simulink model "testrig_susp_knc"  (R2026a)
settings: Solver=ode23t  StopTime=309  MaxStep=0.1  AbsTol=1e-3  EnableMultiTasking=on
PostLoadFcn:
  | Maneuver = MDatabase.KnC.FSAE_Achilles;
  | Visual = sm_car_param_visual('default');
values from neighbouring files (symbols this model uses):
  Vehicle = sm_car_vehcfg_setPeopleOnOff(Vehicle,[0 0 0 0 0],'SuspA1')    [testrig_susp_knc_results.m]
undefined symbols (not defined in the file or in its folder): Axle1D, AxleIn, Init, RaceFix, RaceSpin, X, Y, Z
libraries: fl_lib x12, sm_lib x8, sm_car_testrig_utilities_lib x6, nesl_utility x5, Damper_Element x2, Linkage x1
CloseFcn:
  | clear simlog_sm_car_testrig_quarter_car
  | clear logsout_sm_car_testrig_quarter_car
  | Maneuver = MDatabase.Skidpad.FSAE_Achilles;
Description:
  | Half Car Testrig, Pullrod
  | 
  | Copyright 2021-2024 The MathWorks, Inc.
settings Model: Creator=smiller  LastModifiedBy=andrei
settings SolverCC: MinimalZcImpactIntegration=on
settings DataIOCC: SignalLoggingName=logsout_sm_car_testrig_quarter_car
settings DebuggingCC: ReadBeforeWriteMsg=DisableAll  WriteAfterWriteMsg=DisableAll  WriteAfterReadMsg=DisableAll  MultiTaskDSMMsg=none
settings SFSimCC: SFSimEcho=off
settings SimscapeCC: SimscapeNominalValues="[{\"value\":\"1\",\"unit\":\"A\"},{\"value\":\"1\",\"unit\":\"bar\"},{\"value\":\"1\",\"unit\":\"cm^2\"},{\"value\":\"1\",\"unit\":\"cm^3/s\"},{\"value\":\"1\",\"unit\":\"kJ/kg\"},{\"value\":\"1\",\"unit\":\"kW\"},{\"value\":\"1\",\"unit\":\"l\"},{\"value\":\"1\",\"unit\":\"N\"},{\"value\":\"1\",\"unit\":\"N*m\"},{\"value\":\"1\",\"unit\":\"V\"}]"  SimscapeLogSimulationStatistics=on  SimscapeLogName=simlog_sm_car_testrig_quarter_car  SimscapeLogLimitData=off  SimscapeOperatingPoint=op
settings DiagnosticsConfigSet: SimMechanicsUnconnectedFramePorts=none  SimMechanicsConflictingReferenceFrames=none
settings ExplorerConfigSet: InternalSimMechanicsExplorerSettings=|
  | <ExplorerConfiguration>
  | 
  |   <canonicalview>default</canonicalview>
  | 
  |   <TilePanel>
  |     <TileInfo>
  |       <Tiles Columns="1" Count="1" Height="1112" Rows="1" Width="2985">
  |         <Row Weight="1"/>
  |         <Column Weight="1"/>
  |         <Tile Height="1" Width="1" X="0" Y="0"/>
  |       </Tiles>
  |     </TileInfo>
  |     <SceneInfo>
  |       <SceneViewer>
  |         <IsThisViewStd>
  |           <IsStandardView>off</IsStandardView>
  |           <StandardViewName>Front</StandardViewName>
  |         </IsThisViewStd>
  |         <BGColor>
  |           <R>1</R>
  |           <G>1</G>
  |           <B>1</B>
  |           <A>1</A>
  |         </BGColor>
  |         <Camera>
  |           <DoPerspective>off</DoPerspective>
  |           <Position>
  |             <X>0.57193000000000005</X>
  |             <Y>-0.57911000000000001</Y>
  |             <Z>0.83606000000000003</Z>
  |           </Position>
  |           <Center>
  |             <X>-0.0054200000000000003</X>
  |             <Y>-0.0017600000000000001</Y>
  |             <Z>0.25871</Z>
  |           </Center>
  |           <Up>
  |             <X>-0.40824829046386302</X>
  |             <Y>0.40824829046386302</Y>
  |             <Z>0.81649658092772603</Z>
  |           </Up>
  |           <XLim>0.89132328168650055</XLim>
  |           <YLim>0.71867958298145773</YLim>
  |           <ViewLimDist>0.01</ViewLimDist>
  |         </Camera>
  |       </SceneViewer>
  |     </SceneInfo>
  |   </TilePanel>
  | 
  |   <MechEditorPanel>
  |     <GfxPanelCameraMap/>
  |     <Cameras/>
  |     <VideoCreator>
  |       <IncludeTiles>All</IncludeTiles>
  |       <IncludeTime>on</IncludeTime>
  |       <IncludeWorldFrame>off</IncludeWorldFrame>
  |       <PlaybackSpeedRatio>1</PlaybackSpeedRatio>
  |       <FrameRate>30</FrameRate>
  |       <FrameSize>auto</FrameSize>
  |       <VideoFormat>MotionJPEGAVI</VideoFormat>
  |     </VideoCreator>
  |   </MechEditorPanel>
  | 
  |   <PlaybackSettings>
  |     <PlaybackSpeedFactor>16</PlaybackSpeedFactor>
  |   </PlaybackSettings>
  | 
  | </ExplorerConfiguration>

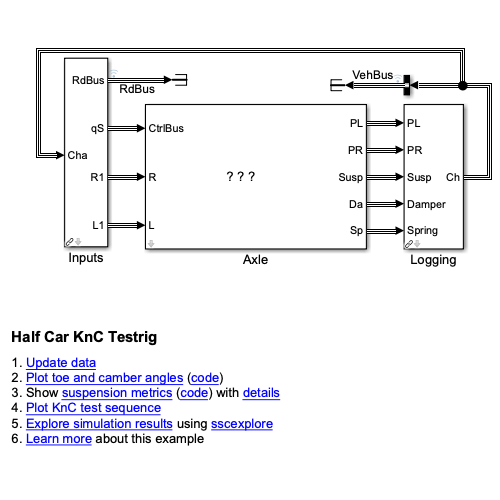
[thumbnail: Simulink's stored preview of the top-level diagram]
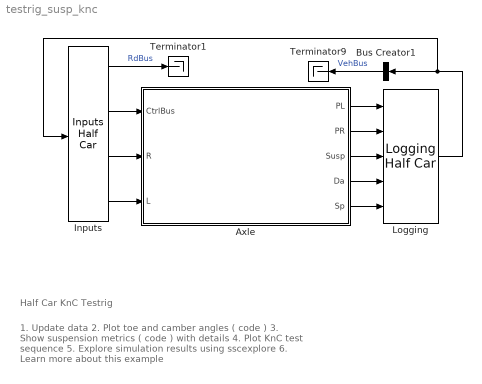
== system testrig_susp_knc ==
  note: Half Car KnC Testrig
  note: 1. Update data
      | 2. Plot toe and camber angles ( code )
      | 3. Show suspension metrics ( code ) with details
      | 4. Plot KnC test sequence
      | 5. Explore simulation results using sscexplore
      | 6. Learn more about this example
  Axle : Subsystem  mask{AxNum=Rear, Vehicle=Vehicle}
      mask prompts: AxNum "Axle"; Vehicle "Vehicle (structure)"
      mask init:
      | curblk = gcb;
      | 
      | AxNumSelection = get_param(curblk,'AxNum');
      | 
      | sWctrSet = sm_car_get_sWheelCentre(Vehicle);
      | 
      | tire_radius = sm_car_vehcfg_getTireRadius(Vehicle);
      | 
      | if strcmp(AxNumSelection,'Front')
      |     axleField = 'Axle1';
      |     suspField = 'SuspA1';
      |     tireField = 'TireA1';
      |     set_param([bdroot '/Inputs'], 'popup_steering_input', 'On');
      |     sWCtr     = sWctrSet(1,:);
      | 
      | else
      |     axleField = 'Axle2';
      |     suspField = 'SuspA2';
      |     tireField = 'TireA2';
      |     set_param([bdroot '/Inputs'], 'popup_steering_input', 'Off');
      |     sWCtr     = sWctrSet(2,:);
      | 
      | end
      | if(strcmp(Vehicle.Chassis.(suspField).class.Value,'Decoupled'))
      |     springLparam = Vehicle.Chassis.Spring.(axleField).Heave;
      |     springLclass = Vehicle.Chassis.Spring.(axleField).Heave.class.Value;
      |     springRparam = Vehicle.Chassis.Spring.(axleField).Roll;
      |     springRclass = Vehicle.Chassis.Spring.(axleField).Roll.class.Value;
      |     damperLparam = Vehicle.Chassis.Damper.(axleField).Heave;
      |     damperLclass = Vehicle.Chassis.Damper.(axleField).Heave.class.Value;
      |     damperRparam = Vehicle.Chassis.Damper.(axleField).Roll;
      |     damperRclass = Vehicle.Chassis.Damper.(axleField).Roll.class.Value;
      | else
      |     springLparam = Vehicle.Chassis.Spring.(axleField);
      |     springLclass = Vehicle.Chassis.Spring.(axleField).class.Value;
      |     springRparam = Vehicle.Chassis.Spring.(axleField);
      |     springRclass = Vehicle.Chassis.Spring.(axleField).class.Value;
      |     damperLparam = Vehicle.Chassis.Damper.(axleField);
      |     damperLclass = Vehicle.Chassis.Damper.(axleField).class.Value;
      |     damperRparam = Vehicle.Chassis.Damper.(axleField);
      |     damperRclass = Vehicle.Chassis.Damper.(axleField).class.Value;
      | end
      mask TypeOptions AxNum: Front | Rear
      mask Display:
      | curblk = gcb;
      | activeVar  = get_param([curblk '/Suspension'],'activevariant');
      | varChoices = get_param([curblk '/Suspension'],'VariantChoices');
      | 
      | varInd = find(strcmp(activeVar,{varChoices(:).Name}));
      | 
      | ActiveVarCmd = get_param(varChoices(varInd).BlockName,'MaskDisplay');
      | eval(ActiveVarCmd);
  Bus Creator1 : BusCreator  Inputs=1
  Inputs : sm_car_testrig_utilities_lib/Inputs Half Car  popup_steering_input=Off
  Logging : sm_car_testrig_utilities_lib/Logging Half Car
  Terminator1 : Terminator
  Terminator9 : Terminator
  wires:
  Bus Creator1/1 -> Terminator9/1  "VehBus"
  Logging/1 -> Inputs/1, Bus Creator1/1
  Inputs/1 -> Terminator1/1  "RdBus"
  Inputs/3 -> Axle/2(R)
  Inputs/4 -> Axle/3(L)
  Inputs/2 -> Axle/1("CtrlBus ")
  Axle/1(PL) -> Logging/1
  Axle/2(PR) -> Logging/2
  Axle/3(Susp) -> Logging/3
  Axle/4(" Da") -> Logging/4
  Axle/5(" Sp") -> Logging/5

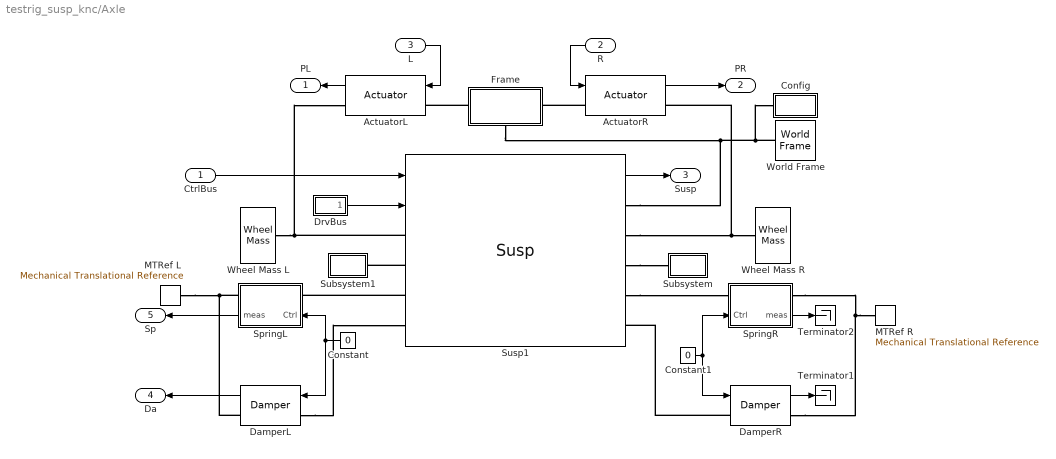
== system testrig_susp_knc/Axle ==
  "CtrlBus " : Inport
  R : Inport  Port=2
  L : Inport  Port=3
  ActuatorL : sm_car_testrig_utilities_lib/Actuator  tire_rad=tire_radius  xCPOffset=Maneuver.xCPOffset
  ActuatorR : sm_car_testrig_utilities_lib/Actuator  tire_rad=tire_radius  xCPOffset=Maneuver.xCPOffset
  Config : Subsystem
  Constant : Constant  Value=0
  Constant1 : Constant  Value=0
  DamperL : Damper_Element/Damper  VariantControl=Variant1  LabelModeActiveChoice=Nonlinear  Damper=damperLparam  VariantLabel=damperLclass
      settings: AttributesFormatString=%<ActiveVariant>
  DamperR : Damper_Element/Damper  VariantControl=Variant1  LabelModeActiveChoice=Nonlinear  Damper=damperRparam  VariantLabel=damperRclass
      settings: AttributesFormatString=%<ActiveVariant>
  DrvBus : Subsystem
  Frame : Subsystem  mask{sWctr=sWCtr}
      mask prompts: sWctr "HP Wheel Center [x y z] (m)"
      settings: PortSchema="{\"entries\":[{\"content\":{\"sides\":[{\"content\":{\"connectorIds\":[\"LConn1\"]},\"type\":\"ConnectorPlacement.EquallySpacedRectSide\",\"uuid\":\"6bafd3c1-bcc7-4e93-aea7-1b45691869cb\"},{\"content\":{\"connectorIds\":[\"RConn1\"],\"side\":\"RIGHT\"},\"type\":\"ConnectorPlacement.EquallySpacedRectSide\",\"uuid\":\"8302b8de-ad89-4cb7-8500-2e46ba409587\"},{\"content\":{\"connectorIds\":[],\"side\":\"TOP\"},\"type\":\"ConnectorPlacement.EquallySpacedRectSide\",\"uuid\":\"64bfca4e-c32f-4ac3-9207-4b63dfa53628\"},{\"content\":{\"connectorIds\":[\"RConn2\"],\"side\":\"BOTTOM\"},\"type\":\"ConnectorPlacement.EquallySpacedRectSide\",\"uuid\":\"4259e7bb-430d-411d-8823-9d547be42692\"}]},\"type\":\"ConnectorPlacement.EquallySpacedConnector\",\"uuid\":\"5df32ab5-9c2e-4acb-a8ad-c01b5f56a7cb\"}],\"packageUris\":[\"http://schema.mathworks.com/mf0/Connector/R2020b\"],\"version\":\"1.0\"}"
  MTRef L : fl_lib/Mechanical/Translational Elements/Mechanical Translational Reference
  MTRef R : fl_lib/Mechanical/Translational Elements/Mechanical Translational Reference
  SpringL : Subsystem  Variant=on  VariantControlMode=label  VariantControl=Variant1  LabelModeActiveChoice=Linear  mask(Variants for Spring){Spring=springLparam, VariantLabel=springLclass}
      mask prompts: Spring "Spring Parameters"; VariantLabel "Variant Label"
      mask help: Select option and provide parameters for spring. Option is chosen by string provided in Variant Label. The parameters for the selected option is contained in Spring data structure.
      mask init:
      | curblk = gcb;
      | 
      | % Set variant for this block 
      | set_param(curblk,'LabelModeActiveChoice',VariantLabel);
      settings: AttributesFormatString=%<ActiveVariant>
      mask Display: disp(' ')
  SpringR : Subsystem  Variant=on  VariantControlMode=label  VariantControl=Variant1  LabelModeActiveChoice=Linear  mask(Variants for Spring){Spring=springRparam, VariantLabel=springRclass}
      mask prompts: Spring "Spring Parameters"; VariantLabel "Variant Label"
      mask help: Select option and provide parameters for spring. Option is chosen by string provided in Variant Label. The parameters for the selected option is contained in Spring data structure.
      mask init:
      | curblk = gcb;
      | 
      | % Set variant for this block 
      | set_param(curblk,'LabelModeActiveChoice',VariantLabel);
      settings: AttributesFormatString=%<ActiveVariant>
      mask Display: disp(' ')
  Subsystem : Subsystem
  Subsystem1 : Subsystem
  Susp1 : Linkage/Susp  VariantControl=Variant1  LabelModeActiveChoice=Linkage  Susp=Vehicle.Chassis.(suspField)  Init=Init.(axleField)  VariantLabel=Vehicle.Chassis.(suspField).class.Value
      settings: AttributesFormatString=%<LabelModeActiveChoice>
  Terminator1 : Terminator
  Terminator2 : Terminator
  Wheel Mass L : sm_car_testrig_utilities_lib/Wheel Mass  tire_param=Vehicle.Chassis.Tire.tirFile.Value
  Wheel Mass R : sm_car_testrig_utilities_lib/Wheel Mass  tire_param=Vehicle.Chassis.Tire.tirFile.Value
  World Frame : sm_lib/Frames and Transforms/World Frame
  PL : Outport
  PR : Outport  Port=2
  Susp : Outport  Port=3
  " Da" : Outport  Port=4
  " Sp" : Outport  Port=5
  wires:
  DamperL/1 -> " Da"/1
  "CtrlBus "/1 -> Susp1/1
  DamperR/1 -> Terminator1/1
  SpringL/1(" meas") -> " Sp"/1
  SpringR/1(" meas") -> Terminator2/1
  ActuatorL/1 -> PL/1
  DrvBus/1(Out1) -> Susp1/2
  Susp1/1 -> Susp/1
  R/1 -> ActuatorR/1
  L/1 -> ActuatorL/1
  ActuatorR/1 -> PR/1
  Constant/1 -> DamperL/1, SpringL/1("Ctrl ")
  Constant1/1 -> DamperR/1, SpringR/1("Ctrl ")
  connections:
  Susp1/RConn3 -- Subsystem/LConn1
  DamperR/LConn1 -- Susp1/RConn5
  World Frame/RConn1 -- Susp1/RConn1 -- Frame/RConn2 -- Config/RConn1
  ActuatorR/RConn1 -- Susp1/RConn2 -- Wheel Mass R/RConn1
  Susp1/LConn3 -- SpringL/LConn1
  Susp1/RConn4 -- SpringR/LConn1
  MTRef L/LConn1 -- DamperL/RConn1 -- SpringL/RConn1
  Wheel Mass L/RConn1 -- Susp1/LConn1 -- ActuatorL/RConn1
  Frame/LConn1 -- ActuatorL/LConn1
  MTRef R/LConn1 -- DamperR/RConn1 -- SpringR/RConn1
  ActuatorR/LConn1 -- Frame/RConn1
  DamperL/LConn1 -- Susp1/LConn4
  Susp1/LConn2 -- Subsystem1/LConn1

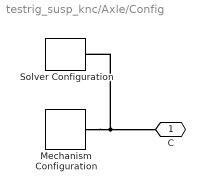
== system testrig_susp_knc/Axle/Config ==
  Mechanism Configuration : sm_lib/Utilities/Mechanism Configuration  UniformGravity=Constant  GravityVector=[0 0 -9.80665]  GravityVectorUnits=m/s^2  LinearizationDelta=0.001  JointModeTransitionNonlinearIterations=2
  Solver Configuration : nesl_utility/Solver Configuration  PhysicalDomain=network_engine_domain  SubClassName=solver  LeftPortType=input  RightPortType=generic  Tones=[]  Harmonics=[]  SimulateNoise=off  Profile=off  UseLocalSampling=off  EnableSwitchedLinearOptims=on  FrequencyDomain=off  UseCCode=off  RelTol=0.001  AbsTol=1e-06  MinStep=1e-09  ToWorkspace=off  RevertToSquareIcSolve=off  NumHomotopyIterations=100  PhasorMode=off  PhasorModeNumHarmonics=1  ConsistencySolver=NEWTON_FTOL  CanonicalOrdering=UNORDERED  OptimizeIntermediates=UNOPTIMIZED  IndexReductionMethod=DerivativeReplacement  DoDC=off  ResidualTolerance=1e-09  ConsistencyTolSource=GLOBAL  ConsistencyAbsTol=0.001  ConsistencyRelTol=0.001  ConsistencyTolFactor=0.001  UseLocalSolver=off  LocalSolverChoice=NE_BACKWARD_EULER_ADVANCER  ResolveIndetEquations=on  FunctionEvalNumThread=1  LocalSolverSampleTime=0.001  DoFixedCost=off  MaxNonlinIter=3  MaxModeIter=2  ComputeImpulses=off  ImpulseIterations=2  LinearAlgebra=Sparse  LinearAlgebraNumThread=0  EquationFormulation=NE_TIME_EF  DelaysMemoryBudget=1024  AutomaticFiltering=on  FilteringTimeConstant=0.001  PartitionStorageMethod=AS_NEEDED  PartitionMemoryBudget=1024  PartitionMethod=FAST  MultibodyUseLocalSolver=off  MultibodyLocalSolverChoice=ODE1  MultibodyLocalSolverSampleTime=0.001
  C : PMIOPort  Side=Right
  connections:
  Mechanism Configuration/RConn1 -- Solver Configuration/RConn1 -- C/RConn1

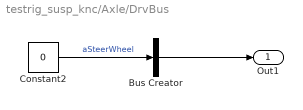
== system testrig_susp_knc/Axle/DrvBus ==
  Bus Creator : BusCreator  Inputs=1
  Constant2 : Constant  Value=0
  Out1 : Outport
  wires:
  Constant2/1 -> Bus Creator/1  "aSteerWheel"
  Bus Creator/1 -> Out1/1

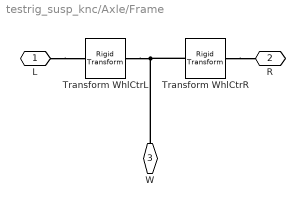
== system testrig_susp_knc/Axle/Frame ==
  Transform WhlCtrL : sm_lib/Frames and Transforms/Rigid Transform  RotationMethod=None  FollAlignAxisA=+X  BaseAlignAxisA=+Y  FollAlignAxisB=+Y  BaseAlignAxisB=+Z  RotationStandardAxis=+Z  RotationAngle=0.0  RotationAngleUnits=deg  RotationArbitraryAxis=[0 0 1]  RotationSequenceAxes=FollowerAxes  RotationSequence=XYX  RotationSequenceAngles=[0 0 0]  RotationSequenceAnglesUnits=deg  RotationMatrix=[1 0 0; 0 1 0; 0 0 1]  Quaternion=[1 0 0 0]  TranslationMethod=Cartesian  TranslationCartesianOffset=sWctr  TranslationCartesianOffsetUnits=m  TranslationStandardAxis=+Z  TranslationStandardOffset=0  TranslationStandardOffsetUnits=m  TranslationROffset=0  TranslationROffsetUnits=m  TranslationThetaOffset=0  TranslationThetaOffsetUnits=deg  TranslationZOffset=0  TranslationZOffsetUnits=m
  Transform WhlCtrR : sm_lib/Frames and Transforms/Rigid Transform  RotationMethod=None  FollAlignAxisA=+X  BaseAlignAxisA=+Y  FollAlignAxisB=+Y  BaseAlignAxisB=+Z  RotationStandardAxis=+Z  RotationAngle=0.0  RotationAngleUnits=deg  RotationArbitraryAxis=[0 0 1]  RotationSequenceAxes=FollowerAxes  RotationSequence=XYX  RotationSequenceAngles=[0 0 0]  RotationSequenceAnglesUnits=deg  RotationMatrix=[1 0 0; 0 1 0; 0 0 1]  Quaternion=[1 0 0 0]  TranslationMethod=Cartesian  TranslationCartesianOffset=sWctr.*[1 -1 1]  TranslationCartesianOffsetUnits=m  TranslationStandardAxis=+Z  TranslationStandardOffset=0  TranslationStandardOffsetUnits=m  TranslationROffset=0  TranslationROffsetUnits=m  TranslationThetaOffset=0  TranslationThetaOffsetUnits=deg  TranslationZOffset=0  TranslationZOffsetUnits=m
  L : PMIOPort  Side=Left
  R : PMIOPort  Port=2  Side=Right
  W : PMIOPort  Port=3  Side=Right
  connections:
  Transform WhlCtrR/LConn1 -- Transform WhlCtrL/LConn1 -- W/RConn1
  L/RConn1 -- Transform WhlCtrL/RConn1
  Transform WhlCtrR/RConn1 -- R/RConn1

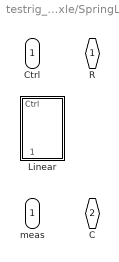
== system testrig_susp_knc/Axle/SpringL ==
  "Ctrl " : Inport
  Linear : Subsystem  VariantControl=Linear  mask(Linear Spring){spr_def0=Spring.xPreload.Value, spr_k=Spring.K.Value, spr_hp_top=Spring.sTop.Value, spr_hp_bot=Spring.sBottom.Value}
      mask prompts: spr_def0 "Spring Preload (m)"; spr_k "Spring Rate (N/m)"; spr_hp_top "HP Top [xyz] (m)"; spr_hp_bot "HP Bottom [xyz] (m)"
      mask help: Spring with linear stiffness.
      mask init:
      | spr_len0 = norm(spr_hp_top-spr_hp_bot);
  " R" : PMIOPort  Side=Left
  " C" : PMIOPort  Port=2  Side=Right
  " meas" : Outport  VectorParamsAs1DForOutWhenUnconnected=off

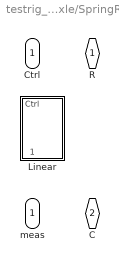
== system testrig_susp_knc/Axle/SpringR ==
  "Ctrl " : Inport
  Linear : Subsystem  VariantControl=Linear  mask(Linear Spring){spr_def0=Spring.xPreload.Value, spr_k=Spring.K.Value, spr_hp_top=Spring.sTop.Value, spr_hp_bot=Spring.sBottom.Value}
      mask prompts: spr_def0 "Spring Preload (m)"; spr_k "Spring Rate (N/m)"; spr_hp_top "HP Top [xyz] (m)"; spr_hp_bot "HP Bottom [xyz] (m)"
      mask help: Spring with linear stiffness.
      mask init:
      | spr_len0 = norm(spr_hp_top-spr_hp_bot);
  " R" : PMIOPort  Side=Left
  " C" : PMIOPort  Port=2  Side=Right
  " meas" : Outport  VectorParamsAs1DForOutWhenUnconnected=off

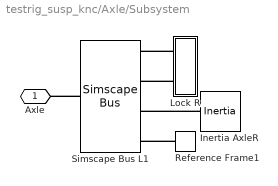
== system testrig_susp_knc/Axle/Subsystem ==
  Inertia AxleR : fl_lib/Mechanical/Rotational Elements/Inertia  inertia=0.01 kg*m^2  num_ports=foundation.enum.numPorts2.one  w_specify=on  w_priority=None  w=0 rad/s  w_nominal_specify=off  w_nominal_value=1  w_nominal_unit=rad/s  t_specify=off  t_priority=None  t=0 N*m  t_nominal_specify=off  t_nominal_value=1  t_nominal_unit=N*m
  Lock R : Subsystem
  Reference Frame1 : sm_lib/Frames and Transforms/Reference Frame
  Simscape Bus L1 : SimscapeBus  HierarchyStrings=RaceSpin;RaceFix;Axle1D;AxleIn
  Axle : PMIOPort  Side=Left
  connections:
  Lock R/LConn2 -- Simscape Bus L1/LConn2
  Reference Frame1/RConn1 -- Simscape Bus L1/LConn4
  Lock R/LConn1 -- Simscape Bus L1/LConn1
  Inertia AxleR/LConn1 -- Simscape Bus L1/LConn3
  Simscape Bus L1/RConn1 -- Axle/RConn1

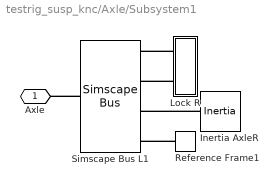
== system testrig_susp_knc/Axle/Subsystem1 ==
  Inertia AxleR : fl_lib/Mechanical/Rotational Elements/Inertia  inertia=0.01 kg*m^2  num_ports=foundation.enum.numPorts2.one  w_specify=on  w_priority=None  w=0 rad/s  w_nominal_specify=off  w_nominal_value=1  w_nominal_unit=rad/s  t_specify=off  t_priority=None  t=0 N*m  t_nominal_specify=off  t_nominal_value=1  t_nominal_unit=N*m
  Lock R : Subsystem
  Reference Frame1 : sm_lib/Frames and Transforms/Reference Frame
  Simscape Bus L1 : SimscapeBus  HierarchyStrings=RaceSpin;RaceFix;Axle1D;AxleIn
  Axle : PMIOPort  Side=Left
  connections:
  Simscape Bus L1/RConn1 -- Axle/RConn1
  Inertia AxleR/LConn1 -- Simscape Bus L1/LConn3
  Lock R/LConn1 -- Simscape Bus L1/LConn1
  Reference Frame1/RConn1 -- Simscape Bus L1/LConn4
  Lock R/LConn2 -- Simscape Bus L1/LConn2

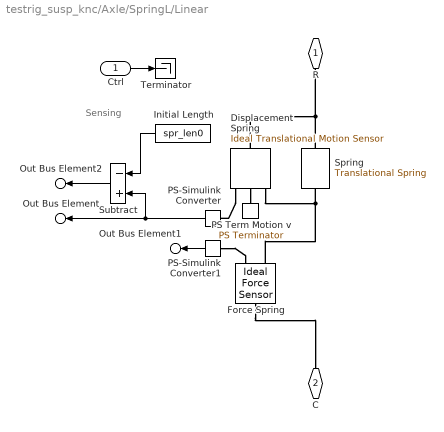
== system testrig_susp_knc/Axle/SpringL/Linear ==
  note: Sensing
  Ctrl : Inport
  Displacement Spring : fl_lib/Mechanical/Mechanical Sensors/Ideal Translational Motion Sensor  reference=foundation.enum.MeasurementReference.difference  acceleration_port=false  velocity_port=true  position_port=true  offset=spr_len0 m
  Force Spring : fl_lib/Mechanical/Mechanical Sensors/Ideal Force Sensor
  Initial Length : Constant  Value=spr_len0
  PS Term Motion v : fl_lib/Physical Signals/Sinks/PS Terminator
  PS-Simulink Converter : nesl_utility/PS-Simulink Converter  PhysicalDomain=network_engine_domain  SubClassName=ps_output  LeftPortType=input  RightPortType=output  PseudoPeriodic=off  Frequencies=[]  VectorFormat=1-D array  Unit=m  AffineConversion=off
  PS-Simulink Converter1 : nesl_utility/PS-Simulink Converter  PhysicalDomain=network_engine_domain  SubClassName=ps_output  LeftPortType=input  RightPortType=output  PseudoPeriodic=off  Frequencies=[]  VectorFormat=1-D array  Unit=N  AffineConversion=off
  Spring : fl_lib/Mechanical/Translational Elements/Translational Spring  spr_rate=spr_k N/m  v_specify=off  v_priority=None  v=0 m/s  v_nominal_specify=off  v_nominal_value=1  v_nominal_unit=m/s  f_specify=off  f_priority=None  f=0 N  f_nominal_specify=off  f_nominal_value=1  f_nominal_unit=N  x_specify=on  x_priority=High  x=-spr_def0 m  x_nominal_specify=off  x_nominal_value=1  x_nominal_unit=m
  Subtract : Sum  Inputs=-+
  Terminator : Terminator
  R : PMIOPort  Side=Left
  C : PMIOPort  Port=2  Side=Right
  Out Bus Element : Outport  VectorParamsAs1DForOutWhenUnconnected=off  PortName=meas  Element=xSpring
  Out Bus Element1 : Outport  VectorParamsAs1DForOutWhenUnconnected=off  PortName=meas  Element=FSpring
  Out Bus Element2 : Outport  VectorParamsAs1DForOutWhenUnconnected=off  PortName=meas  Element=DeltaxSpring
  wires:
  Subtract/1 -> Out Bus Element2/1
  Initial Length/1 -> Subtract/1
  PS-Simulink Converter1/1 -> Out Bus Element1/1
  Ctrl/1 -> Terminator/1
  PS-Simulink Converter/1 -> Subtract/2, Out Bus Element/1
  connections:
  Spring/LConn1 -- R/RConn1 -- Displacement Spring/LConn1
  Spring/RConn1 -- Force Spring/RConn1 -- Displacement Spring/RConn1
  Force Spring/LConn1 -- C/RConn1
  PS-Simulink Converter1/LConn1 -- Force Spring/RConn2
  Displacement Spring/RConn2 -- PS Term Motion v/LConn1
  Displacement Spring/RConn3 -- PS-Simulink Converter/LConn1

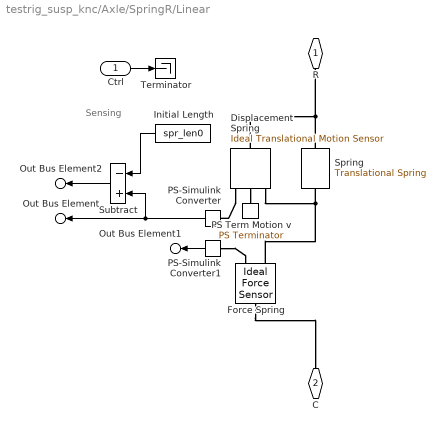
== system testrig_susp_knc/Axle/SpringR/Linear ==
  note: Sensing
  Ctrl : Inport
  Displacement Spring : fl_lib/Mechanical/Mechanical Sensors/Ideal Translational Motion Sensor  reference=foundation.enum.MeasurementReference.difference  acceleration_port=false  velocity_port=true  position_port=true  offset=spr_len0 m
  Force Spring : fl_lib/Mechanical/Mechanical Sensors/Ideal Force Sensor
  Initial Length : Constant  Value=spr_len0
  PS Term Motion v : fl_lib/Physical Signals/Sinks/PS Terminator
  PS-Simulink Converter : nesl_utility/PS-Simulink Converter  PhysicalDomain=network_engine_domain  SubClassName=ps_output  LeftPortType=input  RightPortType=output  PseudoPeriodic=off  Frequencies=[]  VectorFormat=1-D array  Unit=m  AffineConversion=off
  PS-Simulink Converter1 : nesl_utility/PS-Simulink Converter  PhysicalDomain=network_engine_domain  SubClassName=ps_output  LeftPortType=input  RightPortType=output  PseudoPeriodic=off  Frequencies=[]  VectorFormat=1-D array  Unit=N  AffineConversion=off
  Spring : fl_lib/Mechanical/Translational Elements/Translational Spring  spr_rate=spr_k N/m  v_specify=off  v_priority=None  v=0 m/s  v_nominal_specify=off  v_nominal_value=1  v_nominal_unit=m/s  f_specify=off  f_priority=None  f=0 N  f_nominal_specify=off  f_nominal_value=1  f_nominal_unit=N  x_specify=on  x_priority=High  x=-spr_def0 m  x_nominal_specify=off  x_nominal_value=1  x_nominal_unit=m
  Subtract : Sum  Inputs=-+
  Terminator : Terminator
  R : PMIOPort  Side=Left
  C : PMIOPort  Port=2  Side=Right
  Out Bus Element : Outport  VectorParamsAs1DForOutWhenUnconnected=off  PortName=meas  Element=xSpring
  Out Bus Element1 : Outport  VectorParamsAs1DForOutWhenUnconnected=off  PortName=meas  Element=FSpring
  Out Bus Element2 : Outport  VectorParamsAs1DForOutWhenUnconnected=off  PortName=meas  Element=DeltaxSpring
  wires:
  PS-Simulink Converter/1 -> Out Bus Element/1, Subtract/2
  Ctrl/1 -> Terminator/1
  PS-Simulink Converter1/1 -> Out Bus Element1/1
  Initial Length/1 -> Subtract/1
  Subtract/1 -> Out Bus Element2/1
  connections:
  Displacement Spring/RConn3 -- PS-Simulink Converter/LConn1
  Displacement Spring/RConn2 -- PS Term Motion v/LConn1
  PS-Simulink Converter1/LConn1 -- Force Spring/RConn2
  Force Spring/LConn1 -- C/RConn1
  Displacement Spring/RConn1 -- Force Spring/RConn1 -- Spring/RConn1
  Displacement Spring/LConn1 -- R/RConn1 -- Spring/LConn1

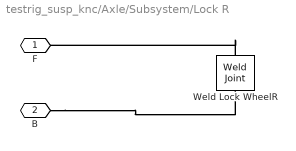
== system testrig_susp_knc/Axle/Subsystem/Lock R ==
  Weld Lock WheelR : sm_lib/Joints/Weld Joint  JointMode=Normal  CompositeWrenchDir=FollowerOnBase  CompositeWrenchFrame=BaseFrame  SenseConstraintForce=off  SenseConstraintTorque=off  SenseTotalForce=off  SenseTotalTorque=off
  F : PMIOPort  Side=Left
  B : PMIOPort  Port=2  Side=Left
  connections:
  Weld Lock WheelR/RConn1 -- F/RConn1
  B/RConn1 -- Weld Lock WheelR/LConn1

== system testrig_susp_knc/Axle/Subsystem1/Lock R ==
  Weld Lock WheelR : sm_lib/Joints/Weld Joint  JointMode=Normal  CompositeWrenchDir=FollowerOnBase  CompositeWrenchFrame=BaseFrame  SenseConstraintForce=off  SenseConstraintTorque=off  SenseTotalForce=off  SenseTotalTorque=off
  F : PMIOPort  Side=Left
  B : PMIOPort  Port=2  Side=Left
  connections:
  B/RConn1 -- Weld Lock WheelR/LConn1
  Weld Lock WheelR/RConn1 -- F/RConn1
